simulink model "sus"  (Simulink 6.5)
settings: Solver=ode45  StartTime=0.0  StopTime=16  RelTol=1e-3
libraries: cdsFilt x266, cdsBitwise x92, cdsEpicsOut x84, cdsEpicsBinIn x56, cdsEpicsIn x20, cdsFiltCtrl x18, cdsMatrix x11, cdsSwitch x7, cdsWD x7, cdsFunctionCall x5, cdsRio1 x4, dac x3
(part 20 of 20)

== system sus/T1/EDCMP/SQRT_BOX ==
  In1 : Inport
  CONST11 : Constant  Value=0
  Choice : Switch  Threshold=1000
  Choice1 : Switch
  Choice2 : Switch  Threshold=1e10
  Choice3 : Switch  Threshold=0.01
  Choice4 : Switch  Threshold=1e-6
  Divide{,1..9} (10 alike) : Product  Inputs=*/  OutScaling=2^-10
  Gain : Gain  Gain=0.05
  Gain{1..10} (10 alike) : Gain  Gain=0.5
  Gain11 : Gain  Gain=0.0001
  Gain12 : Gain  Gain=0.000001
  Gain13 : Gain  Gain=100
  Gain14 : Gain  Gain=10000
  Sum{,1..9} (10 alike) : Sum  Inputs=|++
  Out1 : Outport
  wires:
  Divide/1 -> Sum/1
  Choice1/1 -> Choice/2, Choice2/2, Choice3/2, Choice4/2, Gain/1, Gain13/1, Gain14/1, Divide/1, Divide1/1, Divide2/1, Divide3/1, Divide4/1, Divide5/1, Divide6/1, Divide7/1, Divide8/1, Divide9/1, Gain12/1, Gain11/1
  Gain1/1 -> Sum1/2, Divide1/2
  Divide1/1 -> Sum1/1
  Sum1/1 -> Gain2/1
  Sum/1 -> Gain1/1
  Gain2/1 -> Sum2/2, Divide2/2
  Divide2/1 -> Sum2/1
  Sum2/1 -> Gain4/1
  Gain4/1 -> Sum3/2, Divide3/2
  Divide3/1 -> Sum3/1
  Sum3/1 -> Gain3/1
  Gain3/1 -> Sum4/2, Divide4/2
  Divide4/1 -> Sum4/1
  Sum4/1 -> Gain5/1
  Gain5/1 -> Sum5/2, Divide5/2
  Divide5/1 -> Sum5/1
  Sum5/1 -> Gain6/1
  Gain6/1 -> Sum6/2, Divide6/2
  Divide6/1 -> Sum6/1
  Sum6/1 -> Gain7/1
  Gain7/1 -> Sum7/2, Divide7/2
  Divide7/1 -> Sum7/1
  Sum7/1 -> Gain8/1
  Gain8/1 -> Sum8/2, Divide8/2
  Divide8/1 -> Sum8/1
  Sum8/1 -> Gain9/1
  Gain9/1 -> Sum9/2, Divide9/2
  Divide9/1 -> Sum9/1
  Sum9/1 -> Gain10/1
  Gain10/1 -> Out1/1
  Gain/1 -> Choice/3
  In1/1 -> Choice1/2, Choice1/1
  CONST11/1 -> Choice1/3
  Gain11/1 -> Choice2/3
  Gain12/1 -> Choice2/1
  Choice2/1 -> Choice/1
  Choice/1 -> Choice3/1
  Choice3/1 -> Choice4/1
  Choice4/1 -> Sum/2, Divide/2
  Gain13/1 -> Choice3/3
  Gain14/1 -> Choice4/3

== system sus/T1/EDCMP/SQRT_BOX1 ==
  In1 : Inport
  CONST11 : Constant  Value=0
  Choice : Switch  Threshold=1000
  Choice1 : Switch
  Choice2 : Switch  Threshold=1e10
  Choice3 : Switch  Threshold=0.01
  Choice4 : Switch  Threshold=1e-6
  Divide{,1..9} (10 alike) : Product  Inputs=*/  OutScaling=2^-10
  Gain : Gain  Gain=0.05
  Gain{1..10} (10 alike) : Gain  Gain=0.5
  Gain11 : Gain  Gain=0.0001
  Gain12 : Gain  Gain=0.000001
  Gain13 : Gain  Gain=100
  Gain14 : Gain  Gain=10000
  Sum{,1..9} (10 alike) : Sum  Inputs=|++
  Out1 : Outport
  wires:
  Divide/1 -> Sum/1
  Choice1/1 -> Choice/2, Choice2/2, Choice3/2, Choice4/2, Gain/1, Gain13/1, Gain14/1, Divide/1, Divide1/1, Divide2/1, Divide3/1, Divide4/1, Divide5/1, Divide6/1, Divide7/1, Divide8/1, Divide9/1, Gain12/1, Gain11/1
  Gain1/1 -> Sum1/2, Divide1/2
  Divide1/1 -> Sum1/1
  Sum1/1 -> Gain2/1
  Sum/1 -> Gain1/1
  Gain2/1 -> Sum2/2, Divide2/2
  Divide2/1 -> Sum2/1
  Sum2/1 -> Gain4/1
  Gain4/1 -> Sum3/2, Divide3/2
  Divide3/1 -> Sum3/1
  Sum3/1 -> Gain3/1
  Gain3/1 -> Sum4/2, Divide4/2
  Divide4/1 -> Sum4/1
  Sum4/1 -> Gain5/1
  Gain5/1 -> Sum5/2, Divide5/2
  Divide5/1 -> Sum5/1
  Sum5/1 -> Gain6/1
  Gain6/1 -> Sum6/2, Divide6/2
  Divide6/1 -> Sum6/1
  Sum6/1 -> Gain7/1
  Gain7/1 -> Sum7/2, Divide7/2
  Divide7/1 -> Sum7/1
  Sum7/1 -> Gain8/1
  Gain8/1 -> Sum8/2, Divide8/2
  Divide8/1 -> Sum8/1
  Sum8/1 -> Gain9/1
  Gain9/1 -> Sum9/2, Divide9/2
  Divide9/1 -> Sum9/1
  Sum9/1 -> Gain10/1
  Gain10/1 -> Out1/1
  Gain/1 -> Choice/3
  In1/1 -> Choice1/2, Choice1/1
  CONST11/1 -> Choice1/3
  Gain11/1 -> Choice2/3
  Gain12/1 -> Choice2/1
  Choice2/1 -> Choice/1
  Choice/1 -> Choice3/1
  Choice3/1 -> Choice4/1
  Choice4/1 -> Sum/2, Divide/2
  Gain13/1 -> Choice3/3
  Gain14/1 -> Choice4/3

== system sus/T1/M0/ADD ==
  In1 : Inport
  In2 : Inport  Port=2
  In3 : Inport  Port=3
  In4 : Inport  Port=4
  In5 : Inport  Port=5
  In6 : Inport  Port=6
  In7 : Inport  Port=7
  In8 : Inport  Port=8
  In9 : Inport  Port=9
  In10 : Inport  Port=10
  In11 : Inport  Port=11
  In12 : Inport  Port=12
  Sum{,1..5} (6 alike) : Sum  Inputs=|++
  Out1 : Outport
  Out2 : Outport  Port=2
  Out3 : Outport  Port=3
  Out4 : Outport  Port=4
  Out5 : Outport  Port=5
  Out6 : Outport  Port=6
  wires:
  In1/1 -> Sum/1
  Sum/1 -> Out1/1
  Sum1/1 -> Out2/1
  In2/1 -> Sum1/1
  In3/1 -> Sum2/1
  Sum2/1 -> Out3/1
  Sum3/1 -> Out4/1
  In4/1 -> Sum3/1
  In5/1 -> Sum4/1
  Sum4/1 -> Out5/1
  Sum5/1 -> Out6/1
  In6/1 -> Sum5/1
  In7/1 -> Sum/2
  In8/1 -> Sum1/2
  In9/1 -> Sum2/2
  In10/1 -> Sum3/2
  In11/1 -> Sum4/2
  In12/1 -> Sum5/2

== system sus/T1/M0/BIT ==
  In1 : Inport
  In3 : Inport  Port=2
  In2 : Inport  Port=3
  In4 : Inport  Port=4
  In5 : Inport  Port=5
  In6 : Inport  Port=6
  Constant1 : Constant  Value=4
  Constant2 : Constant  Value=0
  Constant6 : Constant  Value=67108864
  Constant8 : Constant  Value=0
  LogicalOperator10 : Logic  Inputs=12  AllPortsSameDT=off  OutDataTypeMode=Boolean
  Operator{1..12} (12 alike) : RelationalOperator  Operator=~=  LogicOutDataTypeMode=Boolean
  and{1..12} (12 alike) : cdsBitwise/Subsystem  Tag=cdsBitwise  SystemSampleTime=-1
      settings: AttributesFormatString=%<Tag>
  Out1 : Outport
  wires:
  and1/1 -> Operator4/1
  Constant8/1 -> Operator6/2, Operator4/2, Operator1/2, Operator2/2, Operator3/2, Operator5/2
  and4/1 -> Operator1/1
  In1/1 -> and4/1, and10/1
  In3/1 -> and1/1, and7/1
  and2/1 -> Operator2/1
  In2/1 -> and2/1, and8/1
  and3/1 -> Operator3/1
  In4/1 -> and3/1, and9/1
  and5/1 -> Operator5/1
  In5/1 -> and5/1, and11/1
  and6/1 -> Operator6/1
  In6/1 -> and6/1, and12/1
  Constant6/1 -> and4/2, and1/2, and2/2, and3/2, and5/2, and6/2
  and7/1 -> Operator10/1
  Constant2/1 -> Operator12/2, Operator10/2, Operator7/2, Operator8/2, Operator9/2, Operator11/2
  and10/1 -> Operator7/1
  and8/1 -> Operator8/1
  and9/1 -> Operator9/1
  and11/1 -> Operator11/1
  and12/1 -> Operator12/1
  Constant1/1 -> and10/2, and7/2, and8/2, and9/2, and11/2, and12/2
  LogicalOperator10/1 -> Out1/1
  Operator1/1 -> LogicalOperator10/1
  Operator4/1 -> LogicalOperator10/2
  Operator2/1 -> LogicalOperator10/3
  Operator3/1 -> LogicalOperator10/4
  Operator5/1 -> LogicalOperator10/5
  Operator6/1 -> LogicalOperator10/6
  Operator7/1 -> LogicalOperator10/7
  Operator10/1 -> LogicalOperator10/8
  Operator8/1 -> LogicalOperator10/9
  Operator9/1 -> LogicalOperator10/10
  Operator11/1 -> LogicalOperator10/11
  Operator12/1 -> LogicalOperator10/12

== system sus/T1/UCALC/SQRT_BOX ==
  In1 : Inport
  CONST11 : Constant  Value=0
  Choice : Switch  Threshold=1000
  Choice1 : Switch
  Choice2 : Switch  Threshold=1e10
  Choice3 : Switch  Threshold=0.01
  Choice4 : Switch  Threshold=1e-6
  Divide{,1..9} (10 alike) : Product  Inputs=*/  OutScaling=2^-10
  Gain : Gain  Gain=0.05
  Gain{1..10} (10 alike) : Gain  Gain=0.5
  Gain11 : Gain  Gain=0.0001
  Gain12 : Gain  Gain=0.000001
  Gain13 : Gain  Gain=100
  Gain14 : Gain  Gain=10000
  Sum{,1..9} (10 alike) : Sum  Inputs=|++
  Out1 : Outport
  wires:
  Divide/1 -> Sum/1
  Choice1/1 -> Choice/2, Choice2/2, Choice3/2, Choice4/2, Gain/1, Gain13/1, Gain14/1, Divide/1, Divide1/1, Divide2/1, Divide3/1, Divide4/1, Divide5/1, Divide6/1, Divide7/1, Divide8/1, Divide9/1, Gain12/1, Gain11/1
  Gain1/1 -> Sum1/2, Divide1/2
  Divide1/1 -> Sum1/1
  Sum1/1 -> Gain2/1
  Sum/1 -> Gain1/1
  Gain2/1 -> Sum2/2, Divide2/2
  Divide2/1 -> Sum2/1
  Sum2/1 -> Gain4/1
  Gain4/1 -> Sum3/2, Divide3/2
  Divide3/1 -> Sum3/1
  Sum3/1 -> Gain3/1
  Gain3/1 -> Sum4/2, Divide4/2
  Divide4/1 -> Sum4/1
  Sum4/1 -> Gain5/1
  Gain5/1 -> Sum5/2, Divide5/2
  Divide5/1 -> Sum5/1
  Sum5/1 -> Gain6/1
  Gain6/1 -> Sum6/2, Divide6/2
  Divide6/1 -> Sum6/1
  Sum6/1 -> Gain7/1
  Gain7/1 -> Sum7/2, Divide7/2
  Divide7/1 -> Sum7/1
  Sum7/1 -> Gain8/1
  Gain8/1 -> Sum8/2, Divide8/2
  Divide8/1 -> Sum8/1
  Sum8/1 -> Gain9/1
  Gain9/1 -> Sum9/2, Divide9/2
  Divide9/1 -> Sum9/1
  Sum9/1 -> Gain10/1
  Gain10/1 -> Out1/1
  Gain/1 -> Choice/3
  In1/1 -> Choice1/2, Choice1/1
  CONST11/1 -> Choice1/3
  Gain11/1 -> Choice2/3
  Gain12/1 -> Choice2/1
  Choice2/1 -> Choice/1
  Choice/1 -> Choice3/1
  Choice3/1 -> Choice4/1
  Choice4/1 -> Sum/2, Divide/2
  Gain13/1 -> Choice3/3
  Gain14/1 -> Choice4/3

== system sus/T1/UCALC/SQRT_BOX1 ==
  In1 : Inport
  CONST11 : Constant  Value=0
  Choice : Switch  Threshold=1000
  Choice1 : Switch
  Choice2 : Switch  Threshold=1e10
  Choice3 : Switch  Threshold=0.01
  Choice4 : Switch  Threshold=1e-6
  Divide{,1..9} (10 alike) : Product  Inputs=*/  OutScaling=2^-10
  Gain : Gain  Gain=0.05
  Gain{1..10} (10 alike) : Gain  Gain=0.5
  Gain11 : Gain  Gain=0.0001
  Gain12 : Gain  Gain=0.000001
  Gain13 : Gain  Gain=100
  Gain14 : Gain  Gain=10000
  Sum{,1..9} (10 alike) : Sum  Inputs=|++
  Out1 : Outport
  wires:
  Divide/1 -> Sum/1
  Choice1/1 -> Choice/2, Choice2/2, Choice3/2, Choice4/2, Gain/1, Gain13/1, Gain14/1, Divide/1, Divide1/1, Divide2/1, Divide3/1, Divide4/1, Divide5/1, Divide6/1, Divide7/1, Divide8/1, Divide9/1, Gain12/1, Gain11/1
  Gain1/1 -> Sum1/2, Divide1/2
  Divide1/1 -> Sum1/1
  Sum1/1 -> Gain2/1
  Sum/1 -> Gain1/1
  Gain2/1 -> Sum2/2, Divide2/2
  Divide2/1 -> Sum2/1
  Sum2/1 -> Gain4/1
  Gain4/1 -> Sum3/2, Divide3/2
  Divide3/1 -> Sum3/1
  Sum3/1 -> Gain3/1
  Gain3/1 -> Sum4/2, Divide4/2
  Divide4/1 -> Sum4/1
  Sum4/1 -> Gain5/1
  Gain5/1 -> Sum5/2, Divide5/2
  Divide5/1 -> Sum5/1
  Sum5/1 -> Gain6/1
  Gain6/1 -> Sum6/2, Divide6/2
  Divide6/1 -> Sum6/1
  Sum6/1 -> Gain7/1
  Gain7/1 -> Sum7/2, Divide7/2
  Divide7/1 -> Sum7/1
  Sum7/1 -> Gain8/1
  Gain8/1 -> Sum8/2, Divide8/2
  Divide8/1 -> Sum8/1
  Sum8/1 -> Gain9/1
  Gain9/1 -> Sum9/2, Divide9/2
  Divide9/1 -> Sum9/1
  Sum9/1 -> Gain10/1
  Gain10/1 -> Out1/1
  Gain/1 -> Choice/3
  In1/1 -> Choice1/2, Choice1/1
  CONST11/1 -> Choice1/3
  Gain11/1 -> Choice2/3
  Gain12/1 -> Choice2/1
  Choice2/1 -> Choice/1
  Choice/1 -> Choice3/1
  Choice3/1 -> Choice4/1
  Choice4/1 -> Sum/2, Divide/2
  Gain13/1 -> Choice3/3
  Gain14/1 -> Choice4/3

== system sus/T1/UCALC/SQRT_BOX2 ==
  In1 : Inport
  CONST11 : Constant  Value=0
  Choice : Switch  Threshold=1000
  Choice1 : Switch
  Choice2 : Switch  Threshold=1e10
  Choice3 : Switch  Threshold=0.01
  Choice4 : Switch  Threshold=1e-6
  Divide{,1..9} (10 alike) : Product  Inputs=*/  OutScaling=2^-10
  Gain : Gain  Gain=0.05
  Gain{1..10} (10 alike) : Gain  Gain=0.5
  Gain11 : Gain  Gain=0.0001
  Gain12 : Gain  Gain=0.000001
  Gain13 : Gain  Gain=100
  Gain14 : Gain  Gain=10000
  Sum{,1..9} (10 alike) : Sum  Inputs=|++
  Out1 : Outport
  wires:
  Divide/1 -> Sum/1
  Choice1/1 -> Choice/2, Choice2/2, Choice3/2, Choice4/2, Gain/1, Gain13/1, Gain14/1, Divide/1, Divide1/1, Divide2/1, Divide3/1, Divide4/1, Divide5/1, Divide6/1, Divide7/1, Divide8/1, Divide9/1, Gain12/1, Gain11/1
  Gain1/1 -> Sum1/2, Divide1/2
  Divide1/1 -> Sum1/1
  Sum1/1 -> Gain2/1
  Sum/1 -> Gain1/1
  Gain2/1 -> Sum2/2, Divide2/2
  Divide2/1 -> Sum2/1
  Sum2/1 -> Gain4/1
  Gain4/1 -> Sum3/2, Divide3/2
  Divide3/1 -> Sum3/1
  Sum3/1 -> Gain3/1
  Gain3/1 -> Sum4/2, Divide4/2
  Divide4/1 -> Sum4/1
  Sum4/1 -> Gain5/1
  Gain5/1 -> Sum5/2, Divide5/2
  Divide5/1 -> Sum5/1
  Sum5/1 -> Gain6/1
  Gain6/1 -> Sum6/2, Divide6/2
  Divide6/1 -> Sum6/1
  Sum6/1 -> Gain7/1
  Gain7/1 -> Sum7/2, Divide7/2
  Divide7/1 -> Sum7/1
  Sum7/1 -> Gain8/1
  Gain8/1 -> Sum8/2, Divide8/2
  Divide8/1 -> Sum8/1
  Sum8/1 -> Gain9/1
  Gain9/1 -> Sum9/2, Divide9/2
  Divide9/1 -> Sum9/1
  Sum9/1 -> Gain10/1
  Gain10/1 -> Out1/1
  Gain/1 -> Choice/3
  In1/1 -> Choice1/2, Choice1/1
  CONST11/1 -> Choice1/3
  Gain11/1 -> Choice2/3
  Gain12/1 -> Choice2/1
  Choice2/1 -> Choice/1
  Choice/1 -> Choice3/1
  Choice3/1 -> Choice4/1
  Choice4/1 -> Sum/2, Divide/2
  Gain13/1 -> Choice3/3
  Gain14/1 -> Choice4/3

== system sus/T1/UCALC/SQRT_BOX3 ==
  In1 : Inport
  CONST11 : Constant  Value=0
  Choice : Switch  Threshold=1000
  Choice1 : Switch
  Choice2 : Switch  Threshold=1e10
  Choice3 : Switch  Threshold=0.01
  Choice4 : Switch  Threshold=1e-6
  Divide{,1..9} (10 alike) : Product  Inputs=*/  OutScaling=2^-10
  Gain : Gain  Gain=0.05
  Gain{1..10} (10 alike) : Gain  Gain=0.5
  Gain11 : Gain  Gain=0.0001
  Gain12 : Gain  Gain=0.000001
  Gain13 : Gain  Gain=100
  Gain14 : Gain  Gain=10000
  Sum{,1..9} (10 alike) : Sum  Inputs=|++
  Out1 : Outport
  wires:
  Divide/1 -> Sum/1
  Choice1/1 -> Choice/2, Choice2/2, Choice3/2, Choice4/2, Gain/1, Gain13/1, Gain14/1, Divide/1, Divide1/1, Divide2/1, Divide3/1, Divide4/1, Divide5/1, Divide6/1, Divide7/1, Divide8/1, Divide9/1, Gain12/1, Gain11/1
  Gain1/1 -> Sum1/2, Divide1/2
  Divide1/1 -> Sum1/1
  Sum1/1 -> Gain2/1
  Sum/1 -> Gain1/1
  Gain2/1 -> Sum2/2, Divide2/2
  Divide2/1 -> Sum2/1
  Sum2/1 -> Gain4/1
  Gain4/1 -> Sum3/2, Divide3/2
  Divide3/1 -> Sum3/1
  Sum3/1 -> Gain3/1
  Gain3/1 -> Sum4/2, Divide4/2
  Divide4/1 -> Sum4/1
  Sum4/1 -> Gain5/1
  Gain5/1 -> Sum5/2, Divide5/2
  Divide5/1 -> Sum5/1
  Sum5/1 -> Gain6/1
  Gain6/1 -> Sum6/2, Divide6/2
  Divide6/1 -> Sum6/1
  Sum6/1 -> Gain7/1
  Gain7/1 -> Sum7/2, Divide7/2
  Divide7/1 -> Sum7/1
  Sum7/1 -> Gain8/1
  Gain8/1 -> Sum8/2, Divide8/2
  Divide8/1 -> Sum8/1
  Sum8/1 -> Gain9/1
  Gain9/1 -> Sum9/2, Divide9/2
  Divide9/1 -> Sum9/1
  Sum9/1 -> Gain10/1
  Gain10/1 -> Out1/1
  Gain/1 -> Choice/3
  In1/1 -> Choice1/2, Choice1/1
  CONST11/1 -> Choice1/3
  Gain11/1 -> Choice2/3
  Gain12/1 -> Choice2/1
  Choice2/1 -> Choice/1
  Choice/1 -> Choice3/1
  Choice3/1 -> Choice4/1
  Choice4/1 -> Sum/2, Divide/2
  Gain13/1 -> Choice3/3
  Gain14/1 -> Choice4/3

== system sus/T1/VECNORM/SQRT_BOX1 ==
  In1 : Inport
  CONST11 : Constant  Value=0
  Choice : Switch  Threshold=1000
  Choice1 : Switch
  Choice2 : Switch  Threshold=1e10
  Choice3 : Switch  Threshold=0.01
  Choice4 : Switch  Threshold=1e-6
  Divide{,1..9} (10 alike) : Product  Inputs=*/  OutScaling=2^-10
  Gain : Gain  Gain=0.05
  Gain{1..10} (10 alike) : Gain  Gain=0.5
  Gain11 : Gain  Gain=0.0001
  Gain12 : Gain  Gain=0.000001
  Gain13 : Gain  Gain=100
  Gain14 : Gain  Gain=10000
  Sum{,1..9} (10 alike) : Sum  Inputs=|++
  Out1 : Outport
  wires:
  Gain14/1 -> Choice4/3
  Gain13/1 -> Choice3/3
  Choice4/1 -> Divide/2, Sum/2
  Choice3/1 -> Choice4/1
  Choice/1 -> Choice3/1
  Choice2/1 -> Choice/1
  Gain12/1 -> Choice2/1
  Gain11/1 -> Choice2/3
  CONST11/1 -> Choice1/3
  In1/1 -> Choice1/1, Choice1/2
  Gain/1 -> Choice/3
  Gain10/1 -> Out1/1
  Sum9/1 -> Gain10/1
  Divide9/1 -> Sum9/1
  Gain9/1 -> Divide9/2, Sum9/2
  Sum8/1 -> Gain9/1
  Divide8/1 -> Sum8/1
  Gain8/1 -> Divide8/2, Sum8/2
  Sum7/1 -> Gain8/1
  Divide7/1 -> Sum7/1
  Gain7/1 -> Divide7/2, Sum7/2
  Sum6/1 -> Gain7/1
  Divide6/1 -> Sum6/1
  Gain6/1 -> Divide6/2, Sum6/2
  Sum5/1 -> Gain6/1
  Divide5/1 -> Sum5/1
  Gain5/1 -> Divide5/2, Sum5/2
  Sum4/1 -> Gain5/1
  Divide4/1 -> Sum4/1
  Gain3/1 -> Divide4/2, Sum4/2
  Sum3/1 -> Gain3/1
  Divide3/1 -> Sum3/1
  Gain4/1 -> Divide3/2, Sum3/2
  Sum2/1 -> Gain4/1
  Divide2/1 -> Sum2/1
  Gain2/1 -> Divide2/2, Sum2/2
  Sum/1 -> Gain1/1
  Sum1/1 -> Gain2/1
  Divide1/1 -> Sum1/1
  Gain1/1 -> Divide1/2, Sum1/2
  Choice1/1 -> Gain11/1, Gain12/1, Divide9/1, Divide8/1, Divide7/1, Divide6/1, Divide5/1, Divide4/1, Divide3/1, Divide2/1, Divide1/1, Divide/1, Gain14/1, Gain13/1, Gain/1, Choice4/2, Choice3/2, Choice2/2, Choice/2
  Divide/1 -> Sum/1

== system sus/T1/VECNORM/SQRT_BOX2 ==
  In1 : Inport
  CONST11 : Constant  Value=0
  Choice : Switch  Threshold=1000
  Choice1 : Switch
  Choice2 : Switch  Threshold=1e10
  Choice3 : Switch  Threshold=0.01
  Choice4 : Switch  Threshold=1e-6
  Divide{,1..9} (10 alike) : Product  Inputs=*/  OutScaling=2^-10
  Gain : Gain  Gain=0.05
  Gain{1..10} (10 alike) : Gain  Gain=0.5
  Gain11 : Gain  Gain=0.0001
  Gain12 : Gain  Gain=0.000001
  Gain13 : Gain  Gain=100
  Gain14 : Gain  Gain=10000
  Sum{,1..9} (10 alike) : Sum  Inputs=|++
  Out1 : Outport
  wires:
  Gain14/1 -> Choice4/3
  Gain13/1 -> Choice3/3
  Choice4/1 -> Divide/2, Sum/2
  Choice3/1 -> Choice4/1
  Choice/1 -> Choice3/1
  Choice2/1 -> Choice/1
  Gain12/1 -> Choice2/1
  Gain11/1 -> Choice2/3
  CONST11/1 -> Choice1/3
  In1/1 -> Choice1/1, Choice1/2
  Gain/1 -> Choice/3
  Gain10/1 -> Out1/1
  Sum9/1 -> Gain10/1
  Divide9/1 -> Sum9/1
  Gain9/1 -> Divide9/2, Sum9/2
  Sum8/1 -> Gain9/1
  Divide8/1 -> Sum8/1
  Gain8/1 -> Divide8/2, Sum8/2
  Sum7/1 -> Gain8/1
  Divide7/1 -> Sum7/1
  Gain7/1 -> Divide7/2, Sum7/2
  Sum6/1 -> Gain7/1
  Divide6/1 -> Sum6/1
  Gain6/1 -> Divide6/2, Sum6/2
  Sum5/1 -> Gain6/1
  Divide5/1 -> Sum5/1
  Gain5/1 -> Divide5/2, Sum5/2
  Sum4/1 -> Gain5/1
  Divide4/1 -> Sum4/1
  Gain3/1 -> Divide4/2, Sum4/2
  Sum3/1 -> Gain3/1
  Divide3/1 -> Sum3/1
  Gain4/1 -> Divide3/2, Sum3/2
  Sum2/1 -> Gain4/1
  Divide2/1 -> Sum2/1
  Gain2/1 -> Divide2/2, Sum2/2
  Sum/1 -> Gain1/1
  Sum1/1 -> Gain2/1
  Divide1/1 -> Sum1/1
  Gain1/1 -> Divide1/2, Sum1/2
  Choice1/1 -> Gain11/1, Gain12/1, Divide9/1, Divide8/1, Divide7/1, Divide6/1, Divide5/1, Divide4/1, Divide3/1, Divide2/1, Divide1/1, Divide/1, Gain14/1, Gain13/1, Gain/1, Choice4/2, Choice3/2, Choice2/2, Choice/2
  Divide/1 -> Sum/1

== system sus/T1/VECNORM/SQRT_BOX3 ==
  In1 : Inport
  CONST11 : Constant  Value=0
  Choice : Switch  Threshold=1000
  Choice1 : Switch
  Choice2 : Switch  Threshold=1e10
  Choice3 : Switch  Threshold=0.01
  Choice4 : Switch  Threshold=1e-6
  Divide{,1..9} (10 alike) : Product  Inputs=*/  OutScaling=2^-10
  Gain : Gain  Gain=0.05
  Gain{1..10} (10 alike) : Gain  Gain=0.5
  Gain11 : Gain  Gain=0.0001
  Gain12 : Gain  Gain=0.000001
  Gain13 : Gain  Gain=100
  Gain14 : Gain  Gain=10000
  Sum{,1..9} (10 alike) : Sum  Inputs=|++
  Out1 : Outport
  wires:
  Gain14/1 -> Choice4/3
  Gain13/1 -> Choice3/3
  Choice4/1 -> Divide/2, Sum/2
  Choice3/1 -> Choice4/1
  Choice/1 -> Choice3/1
  Choice2/1 -> Choice/1
  Gain12/1 -> Choice2/1
  Gain11/1 -> Choice2/3
  CONST11/1 -> Choice1/3
  In1/1 -> Choice1/1, Choice1/2
  Gain/1 -> Choice/3
  Gain10/1 -> Out1/1
  Sum9/1 -> Gain10/1
  Divide9/1 -> Sum9/1
  Gain9/1 -> Divide9/2, Sum9/2
  Sum8/1 -> Gain9/1
  Divide8/1 -> Sum8/1
  Gain8/1 -> Divide8/2, Sum8/2
  Sum7/1 -> Gain8/1
  Divide7/1 -> Sum7/1
  Gain7/1 -> Divide7/2, Sum7/2
  Sum6/1 -> Gain7/1
  Divide6/1 -> Sum6/1
  Gain6/1 -> Divide6/2, Sum6/2
  Sum5/1 -> Gain6/1
  Divide5/1 -> Sum5/1
  Gain5/1 -> Divide5/2, Sum5/2
  Sum4/1 -> Gain5/1
  Divide4/1 -> Sum4/1
  Gain3/1 -> Divide4/2, Sum4/2
  Sum3/1 -> Gain3/1
  Divide3/1 -> Sum3/1
  Gain4/1 -> Divide3/2, Sum3/2
  Sum2/1 -> Gain4/1
  Divide2/1 -> Sum2/1
  Gain2/1 -> Divide2/2, Sum2/2
  Sum/1 -> Gain1/1
  Sum1/1 -> Gain2/1
  Divide1/1 -> Sum1/1
  Gain1/1 -> Divide1/2, Sum1/2
  Choice1/1 -> Gain11/1, Gain12/1, Divide9/1, Divide8/1, Divide7/1, Divide6/1, Divide5/1, Divide4/1, Divide3/1, Divide2/1, Divide1/1, Divide/1, Gain14/1, Gain13/1, Gain/1, Choice4/2, Choice3/2, Choice2/2, Choice/2
  Divide/1 -> Sum/1
